simulink model "Grid_Islanded_microgrid_final"  (R2019a)
settings: Solver=FixedStepDiscrete  StartTime=0.0  StopTime=10.0  FixedStep=st  RelTol=1e-3
InitFcn:
  | st=5e-6;
  | 
  | P=75e3;
  | V=400;
  | f=50;
  | fsw=5e3;
  | 
  | C_filter=(0.05*P)/(2*pi*f*V^2);
  | %C_filter=9.947e-6
  | 
  | L_filter=(0.1*V^2)/(2*pi*f*P);
  | %L_filter=5.092
  | R_filter=L_filter*100;
undefined symbols (not defined in the file): Ion, Lithium
libraries: powerlib x29, powerlib_meascontrol x9, dspsrcs4 x3, simulink x2, electricdrivelib x1, re_lib x1
settings Model: Creator=dell  LastModifiedBy=dell

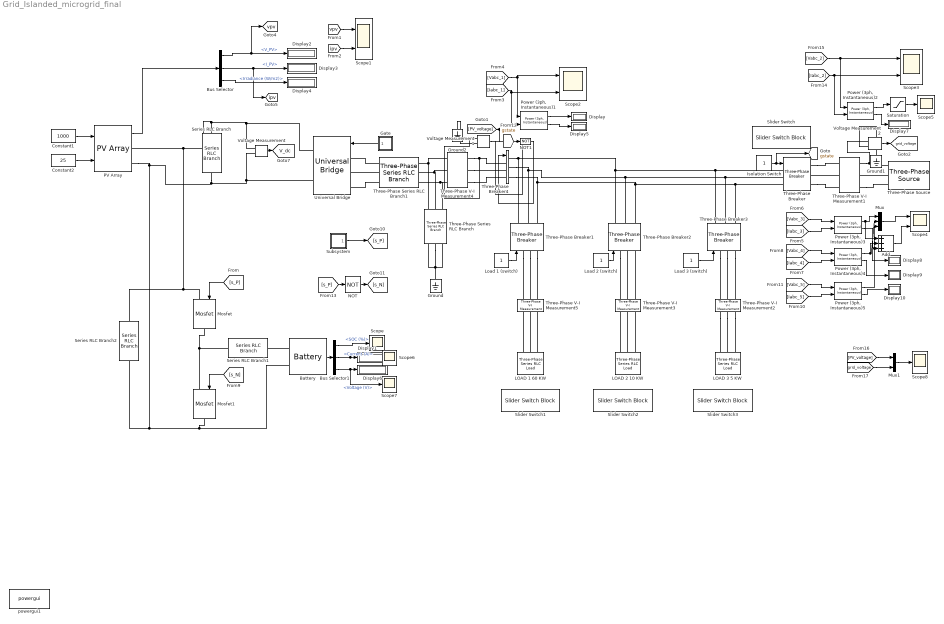
== system Grid_Islanded_microgrid_final ==
  Add : Sum  Inputs=+++
  Battery : electricdrivelib/Extra Sources/Battery  BatType=Lithium-Ion  ShowTempParam=off  ThermalPreset=no  ShowAgeParam=off  NomV=48*9  NomQ=450  SOC=80  Batt_Tr=10e-3  PresetModel=on  MaxQ=450  MinV=324  FullV=502.8424  Dis_rate=195.6522  R=0.0096  Normal_OP=406.9565  expZone="[466.7267       22.1087]"  current=[6.5 13 32.5]  Units=Time  Tci=20  NomT=20  T2=-30  MaxQ2=4.8  FullV2=7.1  Normal_OP2=5.655  expZone2="[6.58           1]"  Rca=0.6  ti=2000  Dp=0  Neq0=0  Tsim=1e6  Ta1=25  Qeol=5.4*0.9  Reol=0.013333*1.2  Char_age=[2.3478, 3]  Dis_age=[2.3478, 10]  N1=1500  N2=10500  N3=1000  N4=1400  Ta2=45  N5=950
      settings: SourceProductName=Simscape Electrical
  Bus Selector : BusSelector  OutputSignals=V_PV,I_PV,Irradiance (W/m2)
  Bus Selector1 : BusSelector  OutputSignals=SOC (%),Current (A),Voltage (V)
  Constant1 : Constant  Value=1000
  Constant2 : Constant  Value=25
  Display{,1..10} (11 alike) : Display
  "Gate " : Subsystem
  Ground : powerlib/Elements/Ground  LConnTagsString=a
      settings: SourceProductName=Simscape Electrical
  Ground1 : powerlib/Elements/Ground  LConnTagsString=a
      settings: SourceProductName=Simscape Electrical
  Ground2 : powerlib/Elements/Ground  LConnTagsString=a
      settings: SourceProductName=Simscape Electrical
  Isolation Switch : Constant
  LOAD 1 60 KW : powerlib/Elements/Three-Phase Series RLC Load  LConnTagsString=A|B|C  Configuration=Y (grounded)  NominalVoltage=400  Vabc=[1e3 1e3 1e3]  Vabcp=[1e3 1e3 1e3]  NominalFrequency=50  UnbalancedPower=off  ActivePower=60e3  InductivePower=0  CapacitivePower=0  Pabc=[10e3 9e3 11e3]  QLabc=[100 90 110]  QCabc=[100 90 110]  Pabcp=[10e3 9e3 11e3]  QLabcp=[100 90 110]  QCabcp=[100 90 110]  Measurements=None  LoadType=constant Z
      settings: SourceProductName=Simscape Electrical
  LOAD 2 10 KW : powerlib/Elements/Three-Phase Series RLC Load  LConnTagsString=A|B|C  Configuration=Y (grounded)  NominalVoltage=400  Vabc=[1e3 1e3 1e3]  Vabcp=[1e3 1e3 1e3]  NominalFrequency=50  UnbalancedPower=off  ActivePower=10e3  InductivePower=0  CapacitivePower=0  Pabc=[10e3 9e3 11e3]  QLabc=[100 90 110]  QCabc=[100 90 110]  Pabcp=[10e3 9e3 11e3]  QLabcp=[100 90 110]  QCabcp=[100 90 110]  Measurements=None  LoadType=constant Z
      settings: SourceProductName=Simscape Electrical
  LOAD 3 5 KW : powerlib/Elements/Three-Phase Series RLC Load  LConnTagsString=A|B|C  Configuration=Y (grounded)  NominalVoltage=400  Vabc=[1e3 1e3 1e3]  Vabcp=[1e3 1e3 1e3]  NominalFrequency=50  UnbalancedPower=off  ActivePower=5e3  InductivePower=0  CapacitivePower=0  Pabc=[10e3 9e3 11e3]  QLabc=[100 90 110]  QCabc=[100 90 110]  Pabcp=[10e3 9e3 11e3]  QLabcp=[100 90 110]  QCabcp=[100 90 110]  Measurements=None  LoadType=constant Z
      settings: SourceProductName=Simscape Electrical
  Load 1 (switch) : Constant
  "Load 2 (switch) " : Constant
  Load 3 (switch) : Constant
  Mosfet : powerlib/Power Electronics/Mosfet  Ron=0.1  Lon=0  Rd=0.01  Vfd=0  IC=0  Rs=1e5  Cs=inf  Measurements=off
      settings: SourceProductName=Simscape Electrical
  Mosfet1 : powerlib/Power Electronics/Mosfet  Ron=0.1  Lon=0  Rd=0.01  Vfd=0  IC=0  Rs=1e5  Cs=inf  Measurements=off
      settings: SourceProductName=Simscape Electrical
  Mux : Mux  Inputs=3
  Mux1 : Mux  Inputs=2
  NOT : Logic  Operator=NOT  IconShape=distinctive  AllPortsSameDT=off  OutDataTypeStr=boolean
  NOT1 : Logic  Operator=NOT  IconShape=distinctive  AllPortsSameDT=off  OutDataTypeStr=boolean
  PV Array : re_lib/Solar/PV Array  Npar=17  Nser=21  PlotType=array @ 1000 W/m2 & specified temperatures  S_vec="[ 1000 900  800  600 400 200 ]"  Temp_C_vec="[ 45 25  ]"  ModuleName=SunPower SPR-E19-245  PlotWhenSelected=off  Pm=245.025  Ncell=72  Voc=48.8  Isc=6.43  Vm=40.5  Im=6.05  beta_Voc_pc=-0.254  alpha_Isc_pc=0.039005  beta_Voc=-0.12395  alpha_Isc=0.002508  IL=6.4383  I0=2.7334e-12  nI=0.92671  Rsh=370.7525  Rs=0.4804  BAL=on  Tc=1e-6  Tfilter=5e-5
      settings: SourceProductName=Simscape Electrical
  Power (3ph, Instantaneous){1..5} (5 alike) : powerlib_meascontrol/Measurements/Power (3ph, Instantaneous)
      settings: SourceProductName=Simscape Electrical
  Saturation : Saturate  UpperLimit=200000
  Scope{,5..8} (5 alike) : Scope
  Scope{1..4} (4 alike) : Scope  NumInputPorts=2
  Series RLC Branch : powerlib/Elements/Series RLC Branch  LConnTagsString=__new0  RConnTagsString=__new0  BranchType=RC  Resistance=1e-3  Inductance=1e-3  SetiL0=off  InitialCurrent=0  Capacitance=1000e-6  Setx0=on  InitialVoltage=1000  Measurements=None
      settings: SourceProductName=Simscape Electrical
  Series RLC Branch1 : powerlib/Elements/Series RLC Branch  LConnTagsString=__new0  RConnTagsString=__new0  BranchType=RL  Resistance=0.05  Inductance=5.76e-4  SetiL0=off  InitialCurrent=0  Capacitance=1e-6  Setx0=off  InitialVoltage=0  Measurements=None
      settings: SourceProductName=Simscape Electrical
  Series RLC Branch2 : powerlib/Elements/Series RLC Branch  LConnTagsString=__new0  RConnTagsString=__new0  BranchType=RC  Resistance=0.195  Inductance=1e-3  SetiL0=off  InitialCurrent=0  Capacitance=500e-6  Setx0=off  InitialVoltage=0  Measurements=None
      settings: SourceProductName=Simscape Electrical
  Slider Switch{,1..3} (4 alike) : SliderSwitchBlock
      settings: Values={{'Off', 'On'}, [0 1]}
  Subsystem : Subsystem
  Three-Phase Series RLC Branch : powerlib/Elements/Three-Phase Series RLC Branch  LConnTagsString=A|B|C  RConnTagsString=A|B|C  BranchType=RC  Resistance=1e-6  Inductance=1e-3  Capacitance=C_filter  Measurements=None
      settings: SourceProductName=Simscape Electrical
  Three-Phase Series RLC Branch1 : powerlib/Elements/Three-Phase Series RLC Branch  LConnTagsString=A|B|C  RConnTagsString=A|B|C  BranchType=RL  Resistance=R_filter  Inductance=L_filter  Capacitance=1e-6  Measurements=None
      settings: SourceProductName=Simscape Electrical
  Three-Phase V-I Measurement1 : powerlib/Measurements/Three-Phase V-I Measurement  VoltageMeasurement=phase-to-phase  SetLabelV=on  LabelV=Vabc_2  Vpu=off  VpuLL=off  CurrentMeasurement=yes  SetLabelI=on  LabelI=Iabc_2  Ipu=off  Pbase=100e6  Vbase=500e3  OutputType=Complex  PhasorSimulation=off  PSBequivalent=0
      settings: SourceProductName=Simscape Electrical
  Three-Phase V-I Measurement2 : powerlib/Measurements/Three-Phase V-I Measurement  VoltageMeasurement=phase-to-ground  SetLabelV=on  LabelV=Vabc_5  Vpu=off  VpuLL=off  CurrentMeasurement=yes  SetLabelI=on  LabelI=Iabc_5  Ipu=off  Pbase=100e6  Vbase=500e3  OutputType=Complex  PhasorSimulation=off  PSBequivalent=0
      settings: SourceProductName=Simscape Electrical
  Three-Phase V-I Measurement3 : powerlib/Measurements/Three-Phase V-I Measurement  VoltageMeasurement=phase-to-ground  SetLabelV=on  LabelV=Vabc_4  Vpu=off  VpuLL=off  CurrentMeasurement=yes  SetLabelI=on  LabelI=Iabc_4  Ipu=off  Pbase=100e6  Vbase=500e3  OutputType=Complex  PhasorSimulation=off  PSBequivalent=0
      settings: SourceProductName=Simscape Electrical
  Three-Phase V-I Measurement4 : powerlib/Measurements/Three-Phase V-I Measurement  VoltageMeasurement=phase-to-phase  SetLabelV=on  LabelV=Vabc_1  Vpu=off  VpuLL=off  CurrentMeasurement=yes  SetLabelI=on  LabelI=Iabc_1  Ipu=off  Pbase=100e6  Vbase=500e3  OutputType=Complex  PhasorSimulation=off  PSBequivalent=0
      settings: SourceProductName=Simscape Electrical
  Three-Phase V-I Measurement5 : powerlib/Measurements/Three-Phase V-I Measurement  VoltageMeasurement=phase-to-ground  SetLabelV=on  LabelV=Vabc_3  Vpu=off  VpuLL=off  CurrentMeasurement=yes  SetLabelI=on  LabelI=Iabc_3  Ipu=off  Pbase=100e6  Vbase=500e3  OutputType=Complex  PhasorSimulation=off  PSBequivalent=0
      settings: SourceProductName=Simscape Electrical
  Three-Phase Breaker{,1..4} (5 alike) : powerlib/Elements/Three-Phase Breaker  InitialState=open  SwitchA=on  SwitchB=on  SwitchC=on  SwitchTimes="[1/60  5/60]"  External=on  BreakerResistance=0.01  SnubberResistance=1e6  SnubberCapacitance=inf  Measurements=None
      settings: SourceProductName=Simscape Electrical
  Three-Phase Source : powerlib/Electrical Sources/Three-Phase Source  InternalConnection=Yg  VoltagePhases=off  Voltage=400  PhaseAngle=0  Voltage_phases=[25e3 25e3 25e3]/sqrt(3)  PhaseAngles_phases=[0 -120 +120]  Frequency=50  NonIdealSource=off  SpecifyImpedance=off  Resistance=0.8929  Inductance=16.58e-3  ShortCircuitLevel=100e6  BaseVoltage=25e3  XRratio=7  BusType=swing  Pref=10e3  Qref=0  Prefabc=[10e3, 10e3, 10e3]  Qrefabc=[0, 0, 0]  Qmin=-inf  Qmax=inf
      settings: SourceProductName=Simscape Electrical
  Universal Bridge : powerlib/Power Electronics/Universal Bridge  Arms=3  SnubberResistance=1e5  SnubberCapacitance=inf  Device=IGBT / Diodes  Ron=1e-3  Lon=0  ForwardVoltages="[  0  0  ]"  ForwardVoltage=0  GTOparameters=[ 10e-6 , 20e-6 ]  IGBTparameters=[ 1e-6 , 2e-6 ]  Measurements=None  Measurements_2=None  converterType=Rectifier
      settings: SourceProductName=Simscape Electrical
  Voltage Measurement : powerlib/Measurements/Voltage Measurement  PhasorSimulation=off  OutputType=Complex  PSBequivalent=0
      settings: SourceProductName=Simscape Electrical
  Voltage Measurement1 : powerlib/Measurements/Voltage Measurement  PhasorSimulation=off  OutputType=Complex  PSBequivalent=0
      settings: SourceProductName=Simscape Electrical
  Voltage Measurement2 : powerlib/Measurements/Voltage Measurement  PhasorSimulation=off  OutputType=Complex  PSBequivalent=0
      settings: SourceProductName=Simscape Electrical
  powergui1 : powerlib/powergui  Priority=1  SimulationMode=Discrete  SampleTime=st  frequency=60  Iterations=50  frequencyindice=0  Pbase=100e6  ErrMax=1e-4  UnitsV=kV  UnitsW=MW  buscounter=0  FunctionMessages=off  echomessages=off  EnableUseOfTLC=off  CurrentSourceSwitches=off  DisableSnubberDevices=off  DisableRonSwitches=off  DisableVfSwitches=off  DisplayEquations=off  AutomaticDiscreteSolvers=off  SolverType=Tustin/Backward Euler (TBE)  Interpol=off  ExternalGateDelay=off  methode=off  Ts=100  x0status=blocks  SPID=on  SwTol=0  HookPort=off  NonlinearTolerance=0  nMaxIteration=15  ContinueOnMaxIteration=off  RestoreLinks=warning  ResistiveCurrentMeasurement=off  Frange=[0:2:500]  Ylog=off  Xlog=on  ShowGrid=off  save=off  variable=ZData  structure=0  ZoomFFT=off  StartTime=0.0  cycles=1  DisplayStyle=1  fundamental=60  FreqAxis=off  MaxFrequency=1000  frequencyindicesteady=1  RmsSteady=1  display=off
      settings: SourceProductName=Simscape Electrical
  tag scope: V_dc=global, grid_voltage=global, gstate=global, ipv=global, vpv=global
  wires:
  Constant2/1 -> PV Array/2
  PV Array/1 -> Bus Selector/1
  Bus Selector/1 -> [vpv], Display2/1  "<V_PV>"
  "Gate "/1(Out1) -> Universal Bridge/1
  Constant1/1 -> PV Array/1
  "Power (3ph, Instantaneous)1"/1 -> Display/1
  Bus Selector/2 -> [ipv], Display3/1  "<I_PV>"
  Bus Selector/3 -> Display4/1  "<Irradiance (W/m2)>"
  Bus Selector1/3 -> Scope7/1, Display6/1  "<Voltage (V)>"
  Bus Selector1/1 -> Scope/1  "<SOC (%)>"
  Battery/1 -> Bus Selector1/1
  Voltage Measurement/1 -> [V_dc]
  Isolation Switch/1 -> [gstate], Three-Phase Breaker/1
  Load 1 (switch)/1 -> Three-Phase Breaker1/1
  "Load 2 (switch) "/1 -> Three-Phase Breaker2/1
  Load 3 (switch)/1 -> Three-Phase Breaker3/1
  [s_P] -> Mosfet/1
  [s_N] -> Mosfet1/1
  [Vabc_2] -> "Power (3ph, Instantaneous)2"/1, Scope3/1
  [Iabc_2] -> "Power (3ph, Instantaneous)2"/2, Scope3/2
  Bus Selector1/2 -> Scope6/1, Display1/1  "<Current (A)>"
  [vpv] -> Scope1/1
  [ipv] -> Scope1/2
  NOT/1 -> [s_N]
  [s_P] -> NOT/1
  Subsystem/1(Out1) -> [s_P]
  [Vabc_1] -> "Power (3ph, Instantaneous)1"/1, Scope2/1
  [Iabc_1] -> "Power (3ph, Instantaneous)1"/2, Scope2/2
  [Iabc_3] -> "Power (3ph, Instantaneous)3"/2
  [Vabc_3] -> "Power (3ph, Instantaneous)3"/1
  [Vabc_4] -> "Power (3ph, Instantaneous)4"/1
  [Iabc_4] -> "Power (3ph, Instantaneous)4"/2
  [Vabc_5] -> "Power (3ph, Instantaneous)5"/1
  [Iabc_5] -> "Power (3ph, Instantaneous)5"/2
  "Power (3ph, Instantaneous)5"/1 -> Add/3, Mux/3
  "Power (3ph, Instantaneous)4"/1 -> Add/2, Mux/2
  [gstate] -> NOT1/1
  NOT1/1 -> Three-Phase Breaker4/1
  Mux/1 -> Scope4/1
  "Power (3ph, Instantaneous)3"/1 -> Add/1, Mux/1
  Add/1 -> Scope4/2
  "Power (3ph, Instantaneous)2"/1 -> Saturation/1
  Voltage Measurement1/1 -> [PV_voltage]
  Mux1/1 -> Scope8/1
  [grid_voltage] -> Mux1/2
  [PV_voltage] -> Mux1/1
  Voltage Measurement2/1 -> [grid_voltage]
  Saturation/1 -> Scope5/1
  "Power (3ph, Instantaneous)1"/2 -> Display5/1
  "Power (3ph, Instantaneous)2"/2 -> Display7/1
  "Power (3ph, Instantaneous)3"/2 -> Display8/1
  "Power (3ph, Instantaneous)4"/2 -> Display9/1
  "Power (3ph, Instantaneous)5"/2 -> Display10/1
  connections:
  Three-Phase V-I Measurement4/LConn3 -- Three-Phase Series RLC Branch/LConn3 -- Three-Phase Series RLC Branch1/RConn3
  Three-Phase V-I Measurement4/LConn1 -- Three-Phase Series RLC Branch1/RConn1 -- Three-Phase Series RLC Branch/LConn1
  Three-Phase V-I Measurement4/LConn2 -- Three-Phase Series RLC Branch1/RConn2 -- Three-Phase Series RLC Branch/LConn2
  Three-Phase Series RLC Branch/RConn1 -- Three-Phase Series RLC Branch/RConn3 -- Ground/LConn1 -- Three-Phase Series RLC Branch/RConn2
  Three-Phase Series RLC Branch1/LConn1 -- Universal Bridge/LConn1
  Three-Phase Series RLC Branch1/LConn3 -- Universal Bridge/LConn3
  Three-Phase Series RLC Branch1/LConn2 -- Universal Bridge/LConn2
  Three-Phase V-I Measurement1/RConn2 -- Three-Phase Breaker/RConn2
  Three-Phase Breaker/RConn1 -- Three-Phase V-I Measurement1/RConn1
  Three-Phase Breaker/RConn3 -- Three-Phase V-I Measurement1/RConn3
  Three-Phase Source/RConn2 -- Three-Phase V-I Measurement1/LConn2
  Three-Phase V-I Measurement1/LConn3 -- Three-Phase Source/RConn3
  Three-Phase V-I Measurement1/LConn1 -- Voltage Measurement2/LConn1 -- Three-Phase Source/RConn1
  Three-Phase V-I Measurement3/LConn2 -- Three-Phase Breaker2/LConn2
  Three-Phase V-I Measurement3/LConn3 -- Three-Phase Breaker2/LConn3
  Three-Phase Breaker2/LConn1 -- Three-Phase V-I Measurement3/LConn1
  LOAD 2 10 KW/LConn2 -- Three-Phase V-I Measurement3/RConn2
  LOAD 2 10 KW/LConn1 -- Three-Phase V-I Measurement3/RConn1
  Three-Phase Breaker3/LConn1 -- Three-Phase V-I Measurement2/LConn1
  Three-Phase Breaker3/LConn2 -- Three-Phase V-I Measurement2/LConn2
  Three-Phase Breaker3/LConn3 -- Three-Phase V-I Measurement2/LConn3
  LOAD 2 10 KW/LConn3 -- Three-Phase V-I Measurement3/RConn3
  LOAD 1 60 KW/LConn1 -- Three-Phase V-I Measurement5/RConn1
  LOAD 1 60 KW/LConn2 -- Three-Phase V-I Measurement5/RConn2
  LOAD 1 60 KW/LConn3 -- Three-Phase V-I Measurement5/RConn3
  Three-Phase V-I Measurement2/RConn3 -- LOAD 3 5 KW/LConn3
  Three-Phase V-I Measurement2/RConn2 -- LOAD 3 5 KW/LConn2
  Three-Phase V-I Measurement2/RConn1 -- LOAD 3 5 KW/LConn1
  Three-Phase Breaker1/LConn1 -- Three-Phase V-I Measurement5/LConn1
  Three-Phase Breaker1/LConn2 -- Three-Phase V-I Measurement5/LConn2
  Three-Phase Breaker1/LConn3 -- Three-Phase V-I Measurement5/LConn3
  Series RLC Branch1/LConn1 -- Mosfet/RConn1 -- Mosfet1/LConn1
  Battery/LConn1 -- Series RLC Branch1/RConn1
  PV Array/RConn1 -- Universal Bridge/RConn1 -- Voltage Measurement/LConn1 -- Series RLC Branch/LConn1 -- Mosfet/LConn1 -- Series RLC Branch2/LConn1
  Mosfet1/RConn1 -- Voltage Measurement/LConn2 -- Universal Bridge/RConn2 -- Series RLC Branch/RConn1 -- PV Array/RConn2 -- Series RLC Branch2/RConn1 -- Battery/LConn2
  Three-Phase Breaker2/RConn2 -- Three-Phase Breaker1/RConn2 -- Three-Phase Breaker4/RConn2 -- Three-Phase Breaker3/RConn2 -- Three-Phase Breaker/LConn2
  Three-Phase Breaker2/RConn3 -- Three-Phase Breaker1/RConn3 -- Three-Phase Breaker4/RConn3 -- Three-Phase Breaker3/RConn3 -- Three-Phase Breaker/LConn3
  Three-Phase Breaker2/RConn1 -- Three-Phase Breaker4/RConn1 -- Three-Phase Breaker1/RConn1 -- Three-Phase Breaker3/RConn1 -- Three-Phase Breaker/LConn1
  Three-Phase V-I Measurement4/RConn1 -- Voltage Measurement1/LConn1 -- Three-Phase Breaker4/LConn1
  Three-Phase V-I Measurement4/RConn2 -- Three-Phase Breaker4/LConn2
  Three-Phase V-I Measurement4/RConn3 -- Three-Phase Breaker4/LConn3
  Ground2/LConn1 -- Voltage Measurement1/LConn2
  Ground1/LConn1 -- Voltage Measurement2/LConn2

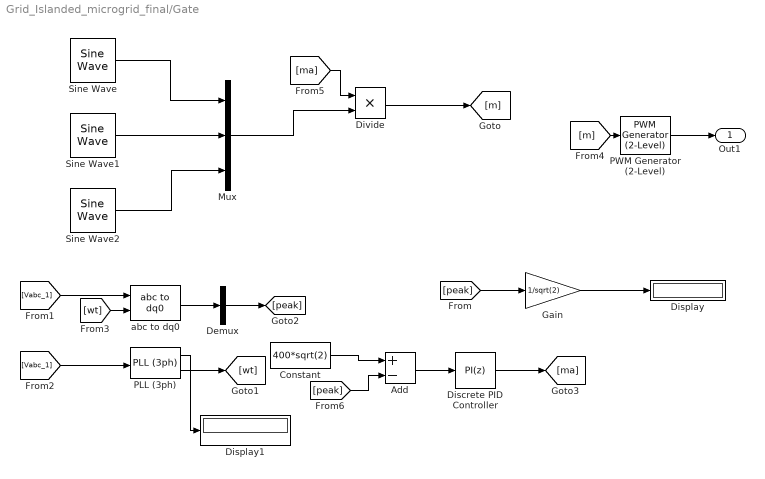
== system Grid_Islanded_microgrid_final/Gate  ==
  Add : Sum  Inputs=+-
  Constant : Constant  Value=400*sqrt(2)
  Demux : Demux  Outputs=1
  Discrete PID Controller : simulink/Continuous/PID Controller  Controller=PI  Form=Parallel  TimeDomain=Discrete-time  SampleTime=st*100  IntegratorMethod=Forward Euler  FilterMethod=Forward Euler  ControllerParametersSource=internal  P=0.001  I=50  D=0  UseFilter=on  N=100  TunerSelectOption=Transfer Function Based (PID Tuner App)  InitialConditionSource=internal  InitialConditionForIntegrator=0  InitialConditionForFilter=0  DifferentiatorICPrevScaledInput=0  ExternalReset=none  TrackingMode=off  Kt=1  LimitOutput=off  UpperSaturationLimit=0.95  LowerSaturationLimit=0.3  LinearizeAsGain=off  AntiWindupMode=none  Kb=1  POutMin=[]  POutMax=[]  IOutMin=[]  IOutMax=[]  DOutMin=[]  DOutMax=[]  NOutMin=[]  NOutMax=[]  SumOutMin=[]  SumOutMax=[]  SaturationOutMin=[]  SaturationOutMax=[]  PParamMin=[]  PParamMax=[]  IParamMin=[]  IParamMax=[]  DParamMin=[]  DParamMax=[]  NParamMin=[]  NParamMax=[]  KbParamMin=[]  KbParamMax=[]  KtParamMin=[]  KtParamMax=[]  KbOutMin=[]  KbOutMax=[]  KtOutMin=[]  KtOutMax=[]  IntegratorOutMin=[]  IntegratorOutMax=[]  FilterOutMin=[]  FilterOutMax=[]  SumI1OutMin=[]  SumI1OutMax=[]  SumI2OutMin=[]  SumI2OutMax=[]  SumI3OutMin=[]  SumI3OutMax=[]  SumI4OutMin=[]  SumI4OutMax=[]  SumDOutMin=[]  SumDOutMax=[]  DifferentiatorOutMin=[]  DifferentiatorOutMax=[]  FilterDiffOutCoefMin=[]  FilterDiffOutCoefMax=[]  ReciprocalOutMin=[]  ReciprocalOutMax=[]  SumDenOutMin=[]  SumDenOutMax=[]  SumNumOutMin=[]  SumNumOutMax=[]  DivideOutMin=[]  DivideOutMax=[]  IntegratorContinuousStateAttributes=''  IntegratorStateMustResolveToSignalObject=off  IntegratorRTWStateStorageClass=Auto  FilterContinuousStateAttributes=''  FilterStateMustResolveToSignalObject=off  FilterRTWStateStorageClass=Auto  ParallelPVariant=InternalParameters  IdealPVariant=Disabled  IVariant=InternalParameters  DVariant=Disabled  IntegratorVariant=Discrete  SatVariant=Disabled  AWVariant=Passthrough  PCopyVariant=Disabled  TRVariant=Disabled  FdbkBlocksVariant=Forward  IdealPFdbkVariant=Disabled  SatFdbkVariant=Disabled  DerivativeFilterVariant=Disabled  NVariant=Disabled  NCopyVariant=Disabled_SignalSpec  FilterICVariant=Disabled  IntegratorICVariant=InternalICs  ExternalResetVariant=Disabled  TRSumVariant=Passthrough  SumFdbkVariant=Disabled  SumVariant=Sum_PI
  Display : Display
  Display1 : Display
  Divide : Product  Inputs=**
  Gain : Gain  Gain=1/sqrt(2)
  Mux : Mux  Inputs=3
  PLL (3ph) : powerlib_meascontrol/PLL/PLL (3ph)  Fmin=45  Par_Init=[0, 50]  ParK=[180, 3200, 1]  TcD=1e-4  MaxRateChangeFreq=12  FilterCutOffFreq=25  Ts=st  AGC=on
      settings: SourceProductName=Simscape Electrical
  PWM Generator (2-Level) : powerlib_meascontrol/Pulse & Signal Generators/PWM Generator (2-Level)  ModulatorType=Three-phase bridge (6 pulses)  ModulatorMode=Unsynchronized  Fc=fsw  Pc=90  nF=27  MinMax="[ -1  1 ]"  SamplingTechnique=Natural  ModulatingSignals=off  m=0.8  Freq=60  Phase=0  Ts=st  ShowCarrierOutport=off
  Sine Wave : dspsrcs4/Sine Wave  Amplitude=1  Frequency=50  Phase=0  SampleMode=Discrete  OutComplex=Real  CompMethod=Trigonometric fcn  TableSize=Speed  SampleTime=st  SamplesPerFrame=1  ResetState=Restart at time zero  OutputFrames=off  dataType=double  wordLen=16  udDataType=sfix(16)  fracBitsMode=Best precision  numFracBits=15  OutDataTypeStr=double  LastOutDataTypeStr=double
  Sine Wave1 : dspsrcs4/Sine Wave  Amplitude=1  Frequency=50  Phase=-2*pi/3  SampleMode=Discrete  OutComplex=Real  CompMethod=Trigonometric fcn  TableSize=Speed  SampleTime=st  SamplesPerFrame=1  ResetState=Restart at time zero  OutputFrames=off  dataType=double  wordLen=16  udDataType=sfix(16)  fracBitsMode=Best precision  numFracBits=15  OutDataTypeStr=double  LastOutDataTypeStr=double
  Sine Wave2 : dspsrcs4/Sine Wave  Amplitude=1  Frequency=50  Phase=2*pi/3  SampleMode=Discrete  OutComplex=Real  CompMethod=Trigonometric fcn  TableSize=Speed  SampleTime=st  SamplesPerFrame=1  ResetState=Restart at time zero  OutputFrames=off  dataType=double  wordLen=16  udDataType=sfix(16)  fracBitsMode=Best precision  numFracBits=15  OutDataTypeStr=double  LastOutDataTypeStr=double
  abc to dq0 : powerlib_meascontrol/Transformations/abc to dq0  Alignment=90 degrees behind phase A axis
      settings: SourceProductName=Simscape Electrical
  Out1 : Outport
  wires:
  Sine Wave2/1 -> Mux/3
  PWM Generator (2-Level)/1 -> Out1/1
  Sine Wave/1 -> Mux/1
  Sine Wave1/1 -> Mux/2
  [ma] -> Divide/1
  Divide/1 -> [m]
  [peak] -> Gain/1
  PLL (3ph)/2 -> [wt]
  Gain/1 -> Display/1
  abc to dq0/1 -> Demux/1
  [Vabc_1] -> PLL (3ph)/1
  [wt] -> abc to dq0/2
  PLL (3ph)/1 -> Display1/1
  Constant/1 -> Add/1
  [peak] -> Add/2
  Add/1 -> Discrete PID Controller/1
  Demux/1 -> [peak]
  Discrete PID Controller/1 -> [ma]
  [Vabc_1] -> abc to dq0/1
  Mux/1 -> Divide/2
  [m] -> PWM Generator (2-Level)/1

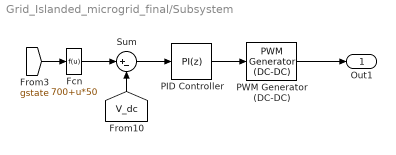
== system Grid_Islanded_microgrid_final/Subsystem ==
  Fcn : Fcn  Expr=700+u*50
  PID Controller : simulink/Continuous/PID Controller  Controller=PI  Form=Parallel  TimeDomain=Discrete-time  SampleTime=st*10  IntegratorMethod=Forward Euler  FilterMethod=Forward Euler  ControllerParametersSource=internal  P=1.5  I=30  D=0  UseFilter=on  N=100  TunerSelectOption=Transfer Function Based (PID Tuner App)  InitialConditionSource=internal  InitialConditionForIntegrator=0  InitialConditionForFilter=0  DifferentiatorICPrevScaledInput=0  ExternalReset=none  TrackingMode=off  Kt=1  LimitOutput=on  UpperSaturationLimit=0.95  LowerSaturationLimit=0  LinearizeAsGain=on  AntiWindupMode=none  Kb=1  POutMin=[]  POutMax=[]  IOutMin=[]  IOutMax=[]  DOutMin=[]  DOutMax=[]  NOutMin=[]  NOutMax=[]  SumOutMin=[]  SumOutMax=[]  SaturationOutMin=[]  SaturationOutMax=[]  PParamMin=[]  PParamMax=[]  IParamMin=[]  IParamMax=[]  DParamMin=[]  DParamMax=[]  NParamMin=[]  NParamMax=[]  KbParamMin=[]  KbParamMax=[]  KtParamMin=[]  KtParamMax=[]  KbOutMin=[]  KbOutMax=[]  KtOutMin=[]  KtOutMax=[]  IntegratorOutMin=[]  IntegratorOutMax=[]  FilterOutMin=[]  FilterOutMax=[]  SumI1OutMin=[]  SumI1OutMax=[]  SumI2OutMin=[]  SumI2OutMax=[]  SumI3OutMin=[]  SumI3OutMax=[]  SumI4OutMin=[]  SumI4OutMax=[]  SumDOutMin=[]  SumDOutMax=[]  DifferentiatorOutMin=[]  DifferentiatorOutMax=[]  FilterDiffOutCoefMin=[]  FilterDiffOutCoefMax=[]  ReciprocalOutMin=[]  ReciprocalOutMax=[]  SumDenOutMin=[]  SumDenOutMax=[]  SumNumOutMin=[]  SumNumOutMax=[]  DivideOutMin=[]  DivideOutMax=[]  IntegratorContinuousStateAttributes=''  IntegratorStateMustResolveToSignalObject=off  IntegratorRTWStateStorageClass=Auto  FilterContinuousStateAttributes=''  FilterStateMustResolveToSignalObject=off  FilterRTWStateStorageClass=Auto  ParallelPVariant=InternalParameters  IdealPVariant=Disabled  IVariant=InternalParameters  DVariant=Disabled  IntegratorVariant=Discrete  SatVariant=Enabled  AWVariant=Passthrough  PCopyVariant=Disabled  TRVariant=Disabled  FdbkBlocksVariant=Forward  IdealPFdbkVariant=Disabled  SatFdbkVariant=Disabled  DerivativeFilterVariant=Disabled  NVariant=Disabled  NCopyVariant=Disabled_SignalSpec  FilterICVariant=Disabled  IntegratorICVariant=InternalICs  ExternalResetVariant=Disabled  TRSumVariant=Passthrough  SumFdbkVariant=Disabled  SumVariant=Sum_PI
  PWM Generator (DC-DC) : powerlib_meascontrol/Pulse & Signal Generators/PWM Generator (DC-DC)  Fsw=fsw  Ts=st
      settings: SourceProductName=Simscape Electrical
  Sum : Sum  Inputs=|+-
  Out1 : Outport
  wires:
  PID Controller/1 -> PWM Generator (DC-DC)/1
  [gstate] -> Fcn/1
  Sum/1 -> PID Controller/1
  [V_dc] -> Sum/2
  PWM Generator (DC-DC)/1 -> Out1/1
  Fcn/1 -> Sum/1
